simulink subsystem "data_counter"  (R2022b)
settings: Solver=VariableStepAuto  StartTime=0.0  StopTime=0.003  RelTol=1e-3
libraries: simulink x5
settings Model: DefaultTestHarness=data_counter_harness  Creator=andre  LastModifiedBy=andre
settings ModelReferenceCC: EnableRefExpFcnMdlSchedulingChecks=on

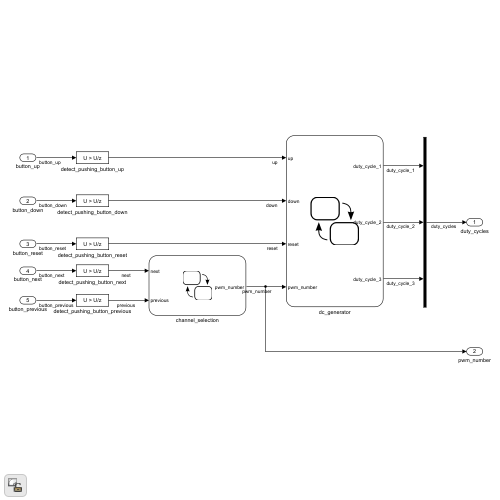
[thumbnail: Simulink's stored preview of the top-level diagram]
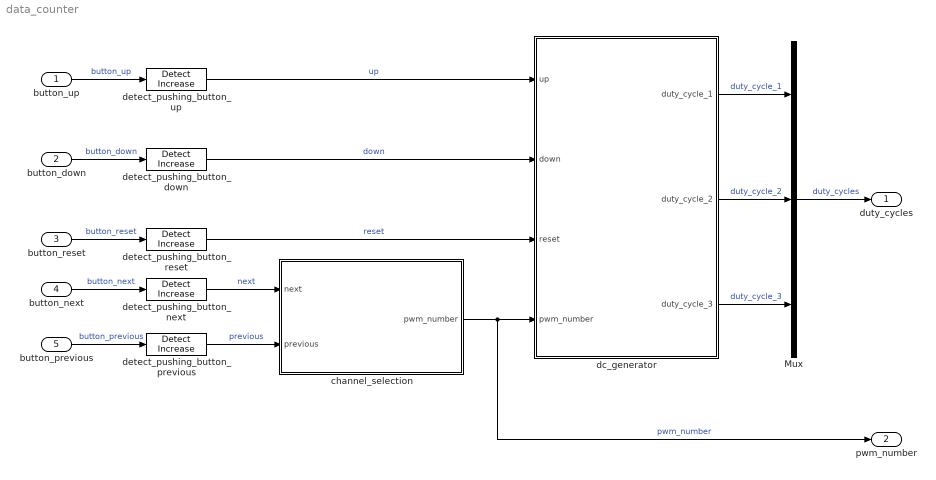
== system data_counter ==
  button_up : Inport  OutDataTypeStr=boolean  PortDimensions=1
  button_down : Inport  Port=2  OutDataTypeStr=boolean  PortDimensions=1
  button_reset : Inport  Port=3  OutDataTypeStr=boolean  PortDimensions=1
  button_next : Inport  Port=4  OutDataTypeStr=boolean  PortDimensions=1
  button_previous : Inport  Port=5  OutDataTypeStr=boolean  PortDimensions=1
  Mux : Mux  Inputs=3
  channel_selection : Stateflow chart  TreatAsAtomicUnit=on
  dc_generator : Stateflow chart  TreatAsAtomicUnit=on
      settings: PortSchema="{\"entries\":[{\"content\":{\"sides\":[{\"content\":{\"connectorIds\":[\"In4\",\"In1\",\"In2\",\"In3\"]},\"type\":\"ConnectorPlacement.EquallySpacedRectSide\",\"uuid\":\"42104dc6-a96b-44e9-8790-f818855c3b17\"},{\"content\":{\"connectorIds\":[\"Out1\",\"Out2\",\"Out3\"],\"side\":\"RIGHT\"},\"type\":\"ConnectorPlacement.EquallySpacedRectSide\",\"uuid\":\"ac049bf6-41b3-4294-b0d6-72eb2b95c579\"},{\"content\":{\"connectorIds\":[],\"side\":\"TOP\"},\"type\":\"ConnectorPlacement.EquallySpacedRectSide\",\"uuid\":\"cb1f105e-f798-4e83-8fed-1a174afd565b\"}]},\"type\":\"ConnectorPlacement.EquallySpacedConnector\",\"uuid\":\"c65f8cfb-24d3-410d-bee6-480d977631af\"}],\"packageUris\":[\"http://schema.mathworks.com/mf0/Connector/R2020b\"],\"version\":\"1.0\"}"
  detect_pushing_button_down : simulink/Logic and Bit Operations/Detect Increase  vinit=0.0  OutDataTypeStr=boolean
  detect_pushing_button_next : simulink/Logic and Bit Operations/Detect Increase  vinit=0.0  OutDataTypeStr=boolean
  detect_pushing_button_previous : simulink/Logic and Bit Operations/Detect Increase  vinit=0.0  OutDataTypeStr=boolean
  detect_pushing_button_reset : simulink/Logic and Bit Operations/Detect Increase  vinit=0.0  OutDataTypeStr=boolean
  detect_pushing_button_up : simulink/Logic and Bit Operations/Detect Increase  vinit=0.0  OutDataTypeStr=boolean
  duty_cycles : Outport  OutDataTypeStr=fixdt(0,SIZE,0)  PortDimensions=3
  pwm_number : Outport  Port=2  OutDataTypeStr=fixdt(0,2,0)  PortDimensions=1
  wires:
  detect_pushing_button_up/1 -> dc_generator/4(up)  "up"
  detect_pushing_button_down/1 -> dc_generator/1(down)  "down"
  detect_pushing_button_reset/1 -> dc_generator/2(reset)  "reset"
  button_up/1 -> detect_pushing_button_up/1  "button_up"
  button_down/1 -> detect_pushing_button_down/1  "button_down"
  button_reset/1 -> detect_pushing_button_reset/1  "button_reset"
  button_next/1 -> detect_pushing_button_next/1  "button_next"
  button_previous/1 -> detect_pushing_button_previous/1  "button_previous"
  detect_pushing_button_previous/1 -> channel_selection/2(previous)  "previous"
  detect_pushing_button_next/1 -> channel_selection/1(next)  "next"
  channel_selection/1(pwm_number) -> dc_generator/3(pwm_number), pwm_number/1  "pwm_number"
  dc_generator/3(duty_cycle_3) -> Mux/3  "duty_cycle_3"
  dc_generator/2(duty_cycle_2) -> Mux/2  "duty_cycle_2"
  dc_generator/1(duty_cycle_1) -> Mux/1  "duty_cycle_1"
  Mux/1 -> duty_cycles/1  "duty_cycles"

== stateflow chart data_counter/channel_selection ==
  settings: executeAtInitialization=1
  state FIRST
    en, du:
    pwm_number = fi(1,0,2,0);
  state SECOND
    en, du:
    pwm_number = fi(2,0,2,0);
  state THIRD
    en, du:
    pwm_number = fi(3,0,2,0);
  (default) -> FIRST
  FIRST -> (junction 12) [order 2] : [previous]
  (junction 19) -> FIRST
  (junction 12) -> (junction 14)
  (junction 17) -> (junction 19)
  FIRST -> SECOND [order 1] : [next]
  SECOND -> FIRST [order 2] : [previous]
  SECOND -> THIRD [order 1] : [next]
  THIRD -> SECOND [order 2] : [previous]
  (junction 14) -> THIRD
  THIRD -> (junction 17) [order 1] : [next]
  data: pwm_number output fixdt(0,2,0) =fi(1,0,2,0); next input boolean; previous input boolean

== stateflow chart data_counter/dc_generator ==
  settings: updateMethod=DISCRETE  sampleTime=1/CLK_FREQ
  state UP
    en:
    if pwm_number == 1
    if duty_cycle_1 >= (2^SIZE-1)
    duty_cycle_1 = fi(2^SIZE-1,0,SIZE,0);
    end
    elseif pwm_number == 2
    if duty_cycle_2 >= (2^SIZE-1)
    duty_cycle_2 = fi(2^SIZE-1,0,SIZE,0);
    end
    else
    if duty_cycle_3 >= (2^SIZE-1)
    duty_cycle_3 = fi(2^SIZE-1,0,SIZE,0);
    end
    end
  state IDLE
    en, du:
    duty_cycle_1 = fi(0,0,SIZE,0);
    duty_cycle_2 = fi(0,0,SIZE,0);
    duty_cycle_3 = fi(0,0,SIZE,0);
  state DOWN
    en:
    if pwm_number == 1
    if duty_cycle_1 < 1
    duty_cycle_1 = fi(0,0,SIZE,0)
    end
    elseif pwm_number == 2
    if duty_cycle_2 < 1
    duty_cycle_2 = fi(0,0,SIZE,0)
    end
    else
    if duty_cycle_3 < 1
    duty_cycle_3 = fi(0,0,SIZE,0)
    end
    end
  (default) -> IDLE
  UP -> (junction 217) [order 2] : [up]
  (junction 217) -> (junction 222) [order 1] : [pwm_number == 1]
  (junction 217) -> (junction 216) [order 2]
  (junction 222) -> (junction 233) : {duty_cycle_1 = fi(duty_cycle_1 + ...
      |  fi(1,0,1,0),0,SIZE,0);}
  UP -> IDLE [order 1] : [reset]
  (junction 216) -> (junction 227) [order 1] : [pwm_number == 2]
  IDLE -> (junction 267) : [up]
  (junction 267) -> (junction 259) [order 1] : [pwm_number == 1]
  (junction 216) -> (junction 218) [order 2] : {duty_cycle_3 = fi(duty_cycle_3 + ...
      |  fi(1,0,1,0),0,SIZE,0);}
  (junction 227) -> (junction 219) : {duty_cycle_2 = fi(duty_cycle_2 + ...
      |  fi(1,0,1,0),0,SIZE,0);}
  (junction 267) -> (junction 266) [order 2]
  (junction 259) -> (junction 258) : {duty_cycle_1 = fi(duty_cycle_1 + ...
      |  fi(1,0,1,0),0,SIZE,0);}
  (junction 266) -> (junction 253) [order 1] : [pwm_number == 2]
  (junction 266) -> (junction 263) [order 2] : {duty_cycle_3 = fi(duty_cycle_3 + ...
      |  fi(1,0,1,0),0,SIZE,0);}
  (junction 253) -> (junction 264) : {duty_cycle_2 = fi(duty_cycle_2 + ...
      |  fi(1,0,1,0),0,SIZE,0);}
  (junction 218) -> UP
  (junction 219) -> (junction 218)
  (junction 233) -> (junction 219)
  (junction 263) -> UP
  UP -> (junction 299) [order 3] : [down]
  (junction 284) -> UP
  (junction 264) -> (junction 263)
  (junction 258) -> (junction 264)
  (junction 288) -> (junction 279) [order 1] : [pwm_number == 1]
  DOWN -> (junction 288) [order 1] : [up]
  (junction 288) -> (junction 287) [order 2]
  (junction 279) -> (junction 278) : {duty_cycle_1 = fi(duty_cycle_1 + ...
      |  fi(1,0,1,0),0,SIZE,0);}
  (junction 287) -> (junction 273) [order 1] : [pwm_number == 2]
  (junction 287) -> (junction 284) [order 2] : {duty_cycle_3 = fi(duty_cycle_3 + ...
      |  fi(1,0,1,0),0,SIZE,0);}
  (junction 273) -> (junction 285) : {duty_cycle_2 = fi(duty_cycle_2 + ...
      |  fi(1,0,1,0),0,SIZE,0);}
  (junction 299) -> (junction 298) [order 1] : [pwm_number == 1]
  (junction 299) -> (junction 302) [order 2]
  (junction 298) -> (junction 300) : {duty_cycle_1 = fi(duty_cycle_1 - ...
      |  fi(1,0,1,0),0,SIZE,0);}
  (junction 285) -> (junction 284)
  (junction 278) -> (junction 285)
  (junction 302) -> (junction 289) [order 1] : [pwm_number == 2]
  (junction 302) -> (junction 296) [order 2] : {duty_cycle_3 = fi(duty_cycle_3 - ...
      |  fi(1,0,1,0),0,SIZE,0);}
  (junction 289) -> (junction 295) : {duty_cycle_2 = fi(duty_cycle_2 - ...
      |  fi(1,0,1,0),0,SIZE,0);}
  DOWN -> IDLE [order 2] : [reset]
  (junction 295) -> (junction 296)
  (junction 300) -> (junction 295)
  (junction 296) -> DOWN
  DOWN -> (junction 251) [order 3] : [down]
  (junction 251) -> (junction 242) [order 1] : [pwm_number == 1]
  (junction 251) -> (junction 250) [order 2]
  (junction 242) -> (junction 241) : {duty_cycle_1 = fi(duty_cycle_1 - ...
      |  fi(1,0,1,0),0,SIZE,0);}
  (junction 250) -> (junction 236) [order 1] : [pwm_number == 2]
  (junction 250) -> (junction 247) [order 2] : {duty_cycle_3 = fi(duty_cycle_3 - ...
      |  fi(1,0,1,0),0,SIZE,0);}
  (junction 236) -> (junction 248) : {duty_cycle_2 = fi(duty_cycle_2 - ...
      |  fi(1,0,1,0),0,SIZE,0);}
  (junction 247) -> DOWN
  (junction 248) -> (junction 247)
  (junction 241) -> (junction 248)
  data: duty_cycle_1 output fixdt(0,SIZE,0) =fi(0,0,SIZE,0); SIZE constant double =SIZE; duty_cycle_2 output fixdt(0,SIZE,0) =fi(0,0,SIZE,0); duty_cycle_3 output fixdt(0,SIZE,0) =fi(0,0,SIZE,0); down input boolean; reset input boolean; pwm_number input; up input
